simulink model "Linear_and_non_Linear"  (R2024a)
settings: Solver=VariableStepAuto  StartTime=0.0  StopTime=10.0  RelTol=1e-3
values from neighbouring files (symbols this model uses):
  J = (m/12)*(l^2*cos(beta)^2+d^2*sin(beta)^2+w^2)    [Group10_Final_Code_Summer.m]    (also in Group10_Final_Main_Code_Winter.m)
  Kd = 5    [Group10_Final_Code_Summer.m]    (also in Group10_Final_Main_Code_Winter.m)
  Kf = 0.07    [Group10_Final_Code_Summer.m]    (also in Group10_Final_Main_Code_Winter.m)
  Kg = 3000    [Group10_Final_Code_Summer.m]    (also in Group10_Final_Main_Code_Winter.m)
  Kp = 0.318    [Group10_Final_Code_Summer.m]    (also in Group10_Final_Main_Code_Winter.m)
  Kt = 0.07    [Group10_Final_Code_Summer.m]    (also in Group10_Final_Main_Code_Winter.m)
  L = 1e-5    (= 1e-05)    [Group10_Final_Code_Summer.m]    (also in Group10_Final_Main_Code_Winter.m)
  R = 10    [Group10_Final_Code_Summer.m]    (also in Group10_Final_Main_Code_Winter.m)
libraries: simulink x2
settings Model: Creator=marin  LastModifiedBy=marin

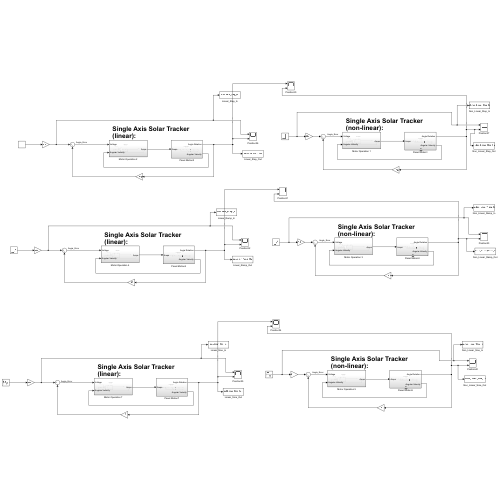
[thumbnail: Simulink's stored preview of the top-level diagram]
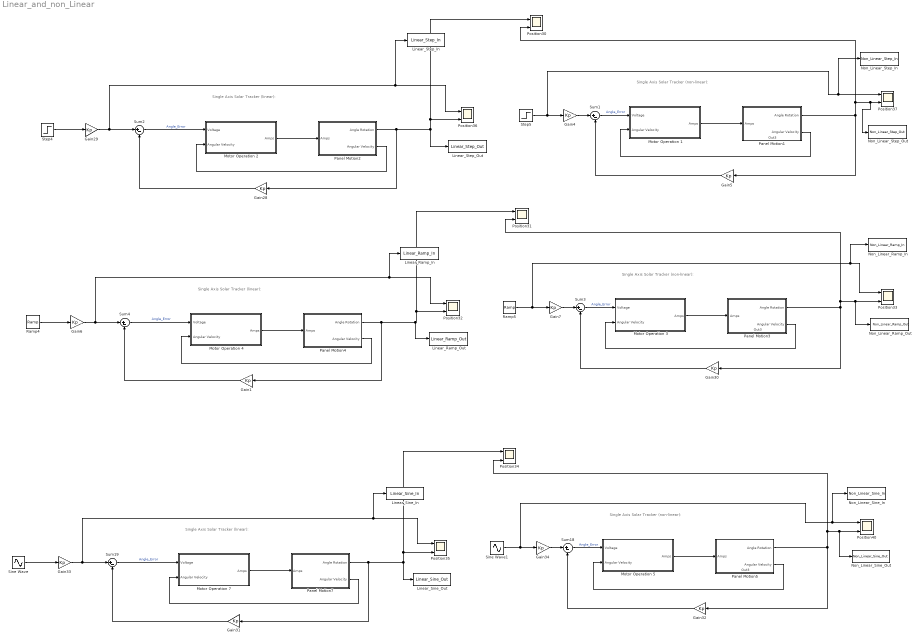
== system Linear_and_non_Linear ==
  note: Single Axis Solar Tracker (linear):
  note: Single Axis Solar Tracker (non-linear):
  note: Single Axis Solar Tracker (non-linear):
  note: Single Axis Solar Tracker (linear):
  note: Single Axis Solar Tracker (linear):
  note: Single Axis Solar Tracker (non-linear):
  Gain{1,4..7,28..34} (12 alike) : Gain  Gain=Kp
  Linear_Ramp_In : ToWorkspace  VariableName=Linear_Ramp_In  SampleTime=-1
  Linear_Ramp_Out : ToWorkspace  VariableName=Linear_Ramp_Out  SampleTime=-1
  Linear_Sine_In : ToWorkspace  VariableName=Linear_Sine_In  SampleTime=-1
  Linear_Sine_Out : ToWorkspace  VariableName=Linear_Sine_Out  SampleTime=-1
  Linear_Step_In : ToWorkspace  VariableName=Linear_Step_In  SampleTime=-1
  Linear_Step_Out : ToWorkspace  VariableName=Linear_Step_Out  SampleTime=-1
  Motor Operation 1 : Subsystem
  Motor Operation 2 : Subsystem
  Motor Operation 3 : Subsystem
  Motor Operation 4 : Subsystem
  Motor Operation 5 : Subsystem
  Motor Operation 7 : Subsystem
  Non_Linear_Ramp_In : ToWorkspace  VariableName=Non_Linear_Ramp_In  SampleTime=-1
  Non_Linear_Ramp_Out : ToWorkspace  VariableName=Non_Linear_Ramp_Out  SampleTime=-1
  Non_Linear_Sine_In : ToWorkspace  VariableName=Non_Linear_Sine_In  SampleTime=-1
  Non_Linear_Sine_Out : ToWorkspace  VariableName=Non_Linear_Sine_Out  SampleTime=-1
  Non_Linear_Step_In : ToWorkspace  VariableName=Non_Linear_Step_In  SampleTime=-1
  Non_Linear_Step_Out : ToWorkspace  VariableName=Non_Linear_Step_Out  SampleTime=-1
  Panel Motion1 : Subsystem
      settings: PortSchema="{\"entries\":[{\"content\":{\"sides\":[{\"content\":{\"connectorIds\":[\"In1\"]},\"type\":\"ConnectorPlacement.EquallySpacedRectSide\",\"uuid\":\"2457b36d-120e-47c4-8d07-640228e5254c\"},{\"content\":{\"connectorIds\":[\"Out1\",\"Out2\"],\"side\":\"RIGHT\"},\"type\":\"ConnectorPlacement.EquallySpacedRectSide\",\"uuid\":\"6776e127-0c13-4a8c-90f1-5ee416f8d651\"},{\"content\":{\"side\":\"TOP\"},\"type\":\"ConnectorPlacement.EquallySpacedRectSide\",\"uuid\":\"01b9375e-d925-43aa-a25a-e625cef73585\"},{\"content\":{\"connectorIds\":[\"Out3\"],\"side\":\"BOTTOM\"},\"type\":\"ConnectorPlacement.EquallySpacedRectSide\",\"uuid\":\"1c8ea06a-a2a0-431e-a15c-ce5bb09036e2\"}]},\"type\":\"ConnectorPlacement.EquallySpacedConnector\",\"uuid\":\"822e0018-41fd-4060-98ab-75615cafefb9\"}],\"packageUris\":[\"http://schema.mathworks.com/mf0/Connector/R2020b\"],\"version\":\"1.0\"}"
  Panel Motion2 : Subsystem
  Panel Motion3 : Subsystem
      settings: PortSchema="{\"entries\":[{\"content\":{\"sides\":[{\"content\":{\"connectorIds\":[\"In1\"]},\"type\":\"ConnectorPlacement.EquallySpacedRectSide\",\"uuid\":\"2457b36d-120e-47c4-8d07-640228e5254c\"},{\"content\":{\"connectorIds\":[\"Out1\",\"Out2\"],\"side\":\"RIGHT\"},\"type\":\"ConnectorPlacement.EquallySpacedRectSide\",\"uuid\":\"6776e127-0c13-4a8c-90f1-5ee416f8d651\"},{\"content\":{\"side\":\"TOP\"},\"type\":\"ConnectorPlacement.EquallySpacedRectSide\",\"uuid\":\"01b9375e-d925-43aa-a25a-e625cef73585\"},{\"content\":{\"connectorIds\":[\"Out3\"],\"side\":\"BOTTOM\"},\"type\":\"ConnectorPlacement.EquallySpacedRectSide\",\"uuid\":\"1c8ea06a-a2a0-431e-a15c-ce5bb09036e2\"}]},\"type\":\"ConnectorPlacement.EquallySpacedConnector\",\"uuid\":\"822e0018-41fd-4060-98ab-75615cafefb9\"}],\"packageUris\":[\"http://schema.mathworks.com/mf0/Connector/R2020b\"],\"version\":\"1.0\"}"
  Panel Motion4 : Subsystem
  Panel Motion5 : Subsystem
      settings: PortSchema="{\"entries\":[{\"content\":{\"sides\":[{\"content\":{\"connectorIds\":[\"In1\"]},\"type\":\"ConnectorPlacement.EquallySpacedRectSide\",\"uuid\":\"2457b36d-120e-47c4-8d07-640228e5254c\"},{\"content\":{\"connectorIds\":[\"Out1\",\"Out2\"],\"side\":\"RIGHT\"},\"type\":\"ConnectorPlacement.EquallySpacedRectSide\",\"uuid\":\"6776e127-0c13-4a8c-90f1-5ee416f8d651\"},{\"content\":{\"side\":\"TOP\"},\"type\":\"ConnectorPlacement.EquallySpacedRectSide\",\"uuid\":\"01b9375e-d925-43aa-a25a-e625cef73585\"},{\"content\":{\"connectorIds\":[\"Out3\"],\"side\":\"BOTTOM\"},\"type\":\"ConnectorPlacement.EquallySpacedRectSide\",\"uuid\":\"1c8ea06a-a2a0-431e-a15c-ce5bb09036e2\"}]},\"type\":\"ConnectorPlacement.EquallySpacedConnector\",\"uuid\":\"822e0018-41fd-4060-98ab-75615cafefb9\"}],\"packageUris\":[\"http://schema.mathworks.com/mf0/Connector/R2020b\"],\"version\":\"1.0\"}"
  Panel Motion7 : Subsystem
  Position{30..37,40} (9 alike) : Scope  NumInputPorts=2
  Ramp4 : simulink/Sources/Ramp  slope=1  start=0  InitialOutput=0
  Ramp5 : simulink/Sources/Ramp  slope=1  start=0  InitialOutput=0
  Sine Wave : Sin  SampleTime=0
  Sine Wave1 : Sin  SampleTime=0
  Step4 : Step  SampleTime=0
  Step5 : Step  SampleTime=0
  Sum{1..4,18..19} (6 alike) : Sum  Inputs=|+-
  wires:
  Sum4/1 -> Motor Operation 4/1(Voltage)  "Angle_Error"
  Ramp4/1 -> Gain6/1
  Sum2/1 -> Motor Operation 2/1(Voltage)  "Angle_Error"
  Sine Wave1/1 -> Non_Linear_Sine_In/1, Position40/1, Gain34/1
  Sum19/1 -> Motor Operation 7/1(Voltage)  "Angle_Error"
  Step5/1 -> Non_Linear_Step_In/1, Position37/1, Gain4/1
  Sine Wave/1 -> Gain33/1
  Sum3/1 -> Motor Operation 3/1(Voltage)  "Angle_Error"
  Panel Motion1/2(Angular Velocity) -> Motor Operation 1/2(Angular Velocity)
  Ramp5/1 -> Gain7/1, Non_Linear_Ramp_In/1, Position33/1
  Gain1/1 -> Sum4/2
  Gain7/1 -> Sum3/1
  Motor Operation 1/1(Amps) -> Panel Motion1/1(Amps)
  Gain5/1 -> Sum1/2
  Gain4/1 -> Sum1/1
  Panel Motion3/1(Angle Rotation) -> Position31/2, Non_Linear_Ramp_Out/1, Position33/2, Gain30/1
  Panel Motion1/1(Angle Rotation) -> Gain5/1, Position30/2, Non_Linear_Step_Out/1, Position37/2
  Gain29/1 -> Sum2/1, Linear_Step_In/1, Position36/1
  Panel Motion4/2(Angular Velocity) -> Motor Operation 4/2(Angular Velocity)
  Sum18/1 -> Motor Operation 5/1(Voltage)  "Angle_Error"
  Panel Motion4/1(Angle Rotation) -> Linear_Ramp_Out/1, Position32/2, Position31/1, Gain1/1
  Panel Motion5/1(Angle Rotation) -> Gain32/1, Position34/2, Non_Linear_Sine_Out/1, Position40/2
  Panel Motion2/1(Angle Rotation) -> Gain28/1, Position30/1, Position36/2, Linear_Step_Out/1
  Motor Operation 2/1(Amps) -> Panel Motion2/1(Amps)
  Panel Motion3/2(Angular Velocity) -> Motor Operation 3/2(Angular Velocity)
  Panel Motion7/2(Angular Velocity) -> Motor Operation 7/2(Angular Velocity)
  Motor Operation 3/1(Amps) -> Panel Motion3/1(Amps)
  Motor Operation 7/1(Amps) -> Panel Motion7/1(Amps)
  Gain34/1 -> Sum18/1
  Gain6/1 -> Linear_Ramp_In/1, Position32/1, Sum4/1
  Panel Motion5/2(Angular Velocity) -> Motor Operation 5/2(Angular Velocity)
  Gain32/1 -> Sum18/2
  Motor Operation 4/1(Amps) -> Panel Motion4/1(Amps)
  Step4/1 -> Gain29/1
  Gain31/1 -> Sum19/2
  Sum1/1 -> Motor Operation 1/1(Voltage)  "Angle_Error"
  Motor Operation 5/1(Amps) -> Panel Motion5/1(Amps)
  Gain28/1 -> Sum2/2
  Gain33/1 -> Sum19/1, Linear_Sine_In/1, Position35/1
  Panel Motion2/2(Angular Velocity) -> Motor Operation 2/2(Angular Velocity)
  Gain30/1 -> Sum3/2
  Panel Motion7/1(Angle Rotation) -> Gain31/1, Linear_Sine_Out/1, Position34/1, Position35/2

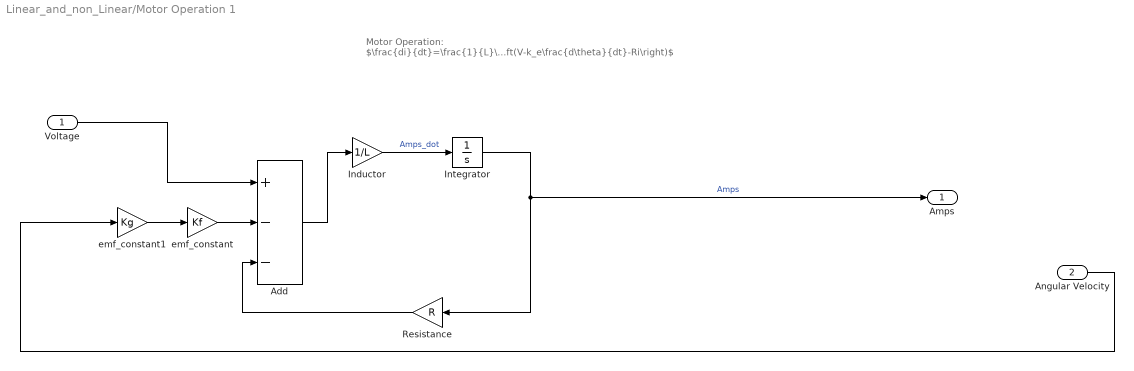
== system Linear_and_non_Linear/Motor Operation 1 ==
  note: Motor Operation:
      | $\frac{di}{dt}=\frac{1}{L}\left(V-k_e\frac{d\theta}{dt}-Ri\right)$
  Voltage : Inport
  Angular Velocity : Inport  Port=2
  Add : Sum  Inputs=+--
  Inductor : Gain  Gain=1/L
  Integrator : Integrator
  Resistance : Gain  Gain=R
  emf_constant : Gain  Gain=Kf
  emf_constant1 : Gain  Gain=Kg
  Amps : Outport
  wires:
  emf_constant/1 -> Add/2
  Resistance/1 -> Add/3
  Add/1 -> Inductor/1
  Inductor/1 -> Integrator/1  "Amps_dot"
  Angular Velocity/1 -> emf_constant1/1
  Voltage/1 -> Add/1
  Integrator/1 -> Resistance/1, Amps/1  "Amps"
  emf_constant1/1 -> emf_constant/1

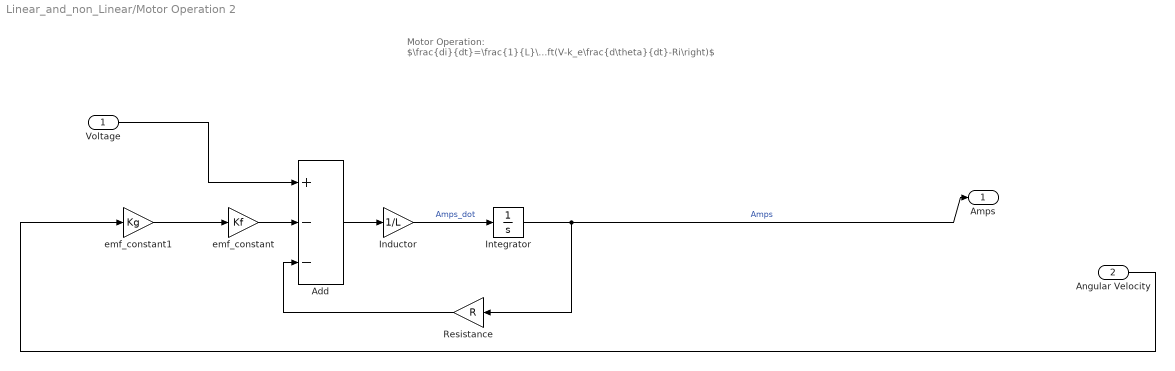
== system Linear_and_non_Linear/Motor Operation 2 ==
  note: Motor Operation:
      | $\frac{di}{dt}=\frac{1}{L}\left(V-k_e\frac{d\theta}{dt}-Ri\right)$
  Voltage : Inport
  Angular Velocity : Inport  Port=2
  Add : Sum  Inputs=+--
  Inductor : Gain  Gain=1/L
  Integrator : Integrator
  Resistance : Gain  Gain=R
  emf_constant : Gain  Gain=Kf
  emf_constant1 : Gain  Gain=Kg
  Amps : Outport
  wires:
  emf_constant/1 -> Add/2
  Resistance/1 -> Add/3
  Add/1 -> Inductor/1
  Inductor/1 -> Integrator/1  "Amps_dot"
  Angular Velocity/1 -> emf_constant1/1
  Voltage/1 -> Add/1
  Integrator/1 -> Amps/1, Resistance/1  "Amps"
  emf_constant1/1 -> emf_constant/1

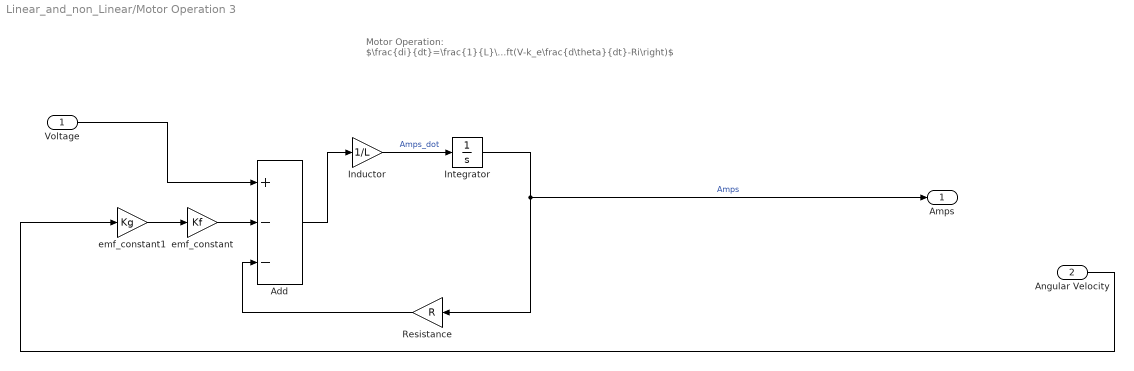
== system Linear_and_non_Linear/Motor Operation 3 ==
  note: Motor Operation:
      | $\frac{di}{dt}=\frac{1}{L}\left(V-k_e\frac{d\theta}{dt}-Ri\right)$
  Voltage : Inport
  Angular Velocity : Inport  Port=2
  Add : Sum  Inputs=+--
  Inductor : Gain  Gain=1/L
  Integrator : Integrator
  Resistance : Gain  Gain=R
  emf_constant : Gain  Gain=Kf
  emf_constant1 : Gain  Gain=Kg
  Amps : Outport
  wires:
  emf_constant1/1 -> emf_constant/1
  Integrator/1 -> Amps/1, Resistance/1  "Amps"
  Voltage/1 -> Add/1
  Angular Velocity/1 -> emf_constant1/1
  Inductor/1 -> Integrator/1  "Amps_dot"
  Add/1 -> Inductor/1
  Resistance/1 -> Add/3
  emf_constant/1 -> Add/2

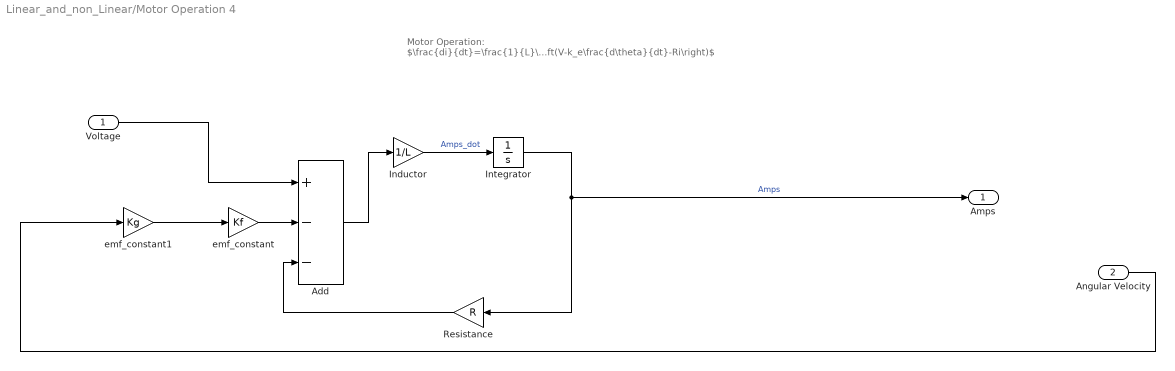
== system Linear_and_non_Linear/Motor Operation 4 ==
  note: Motor Operation:
      | $\frac{di}{dt}=\frac{1}{L}\left(V-k_e\frac{d\theta}{dt}-Ri\right)$
  Voltage : Inport
  Angular Velocity : Inport  Port=2
  Add : Sum  Inputs=+--
  Inductor : Gain  Gain=1/L
  Integrator : Integrator
  Resistance : Gain  Gain=R
  emf_constant : Gain  Gain=Kf
  emf_constant1 : Gain  Gain=Kg
  Amps : Outport
  wires:
  emf_constant1/1 -> emf_constant/1
  Integrator/1 -> Amps/1, Resistance/1  "Amps"
  Voltage/1 -> Add/1
  Angular Velocity/1 -> emf_constant1/1
  Inductor/1 -> Integrator/1  "Amps_dot"
  Add/1 -> Inductor/1
  Resistance/1 -> Add/3
  emf_constant/1 -> Add/2

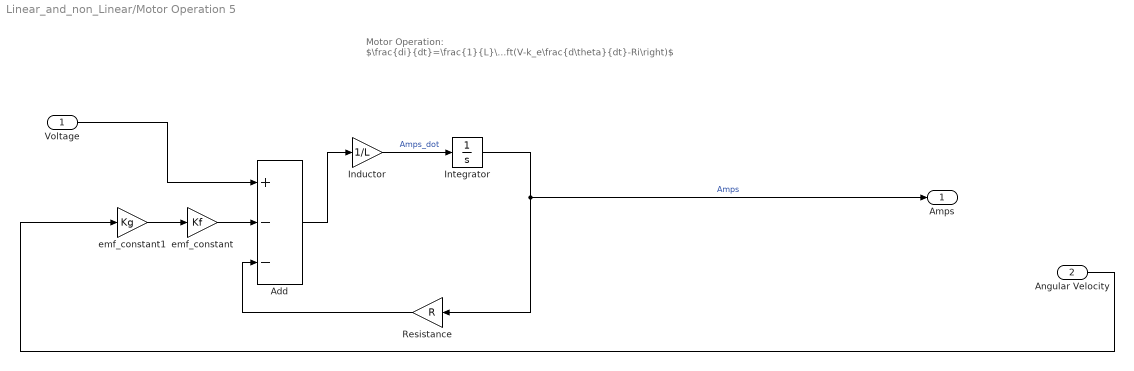
== system Linear_and_non_Linear/Motor Operation 5 ==
  note: Motor Operation:
      | $\frac{di}{dt}=\frac{1}{L}\left(V-k_e\frac{d\theta}{dt}-Ri\right)$
  Voltage : Inport
  Angular Velocity : Inport  Port=2
  Add : Sum  Inputs=+--
  Inductor : Gain  Gain=1/L
  Integrator : Integrator
  Resistance : Gain  Gain=R
  emf_constant : Gain  Gain=Kf
  emf_constant1 : Gain  Gain=Kg
  Amps : Outport
  wires:
  emf_constant/1 -> Add/2
  Resistance/1 -> Add/3
  Add/1 -> Inductor/1
  Inductor/1 -> Integrator/1  "Amps_dot"
  Angular Velocity/1 -> emf_constant1/1
  Voltage/1 -> Add/1
  Integrator/1 -> Resistance/1, Amps/1  "Amps"
  emf_constant1/1 -> emf_constant/1

== system Linear_and_non_Linear/Motor Operation 7 ==
  note: Motor Operation:
      | $\frac{di}{dt}=\frac{1}{L}\left(V-k_e\frac{d\theta}{dt}-Ri\right)$
  Voltage : Inport
  Angular Velocity : Inport  Port=2
  Add : Sum  Inputs=+--
  Inductor : Gain  Gain=1/L
  Integrator : Integrator
  Resistance : Gain  Gain=R
  emf_constant : Gain  Gain=Kf
  emf_constant1 : Gain  Gain=Kg
  Amps : Outport
  wires:
  emf_constant/1 -> Add/2
  Resistance/1 -> Add/3
  Add/1 -> Inductor/1
  Inductor/1 -> Integrator/1  "Amps_dot"
  Angular Velocity/1 -> emf_constant1/1
  Voltage/1 -> Add/1
  Integrator/1 -> Resistance/1, Amps/1  "Amps"
  emf_constant1/1 -> emf_constant/1

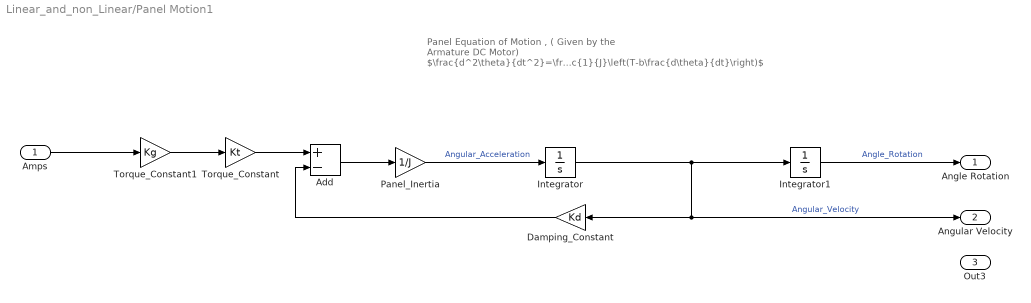
== system Linear_and_non_Linear/Panel Motion1 ==
  note: Panel Equation of Motion ,
      | ( Given by the Armature DC Motor)
      | $\frac{d^2\theta}{dt^2}=\frac{1}{J}\left(T-b\frac{d\theta}{dt}\right)$
  Amps : Inport
  Add : Sum  Inputs=+-
  Damping_Constant : Gain  Gain=Kd
  Integrator : Integrator
  Integrator1 : Integrator
  Panel_Inertia : Gain  Gain=1/J
  Torque_Constant : Gain  Gain=Kt
  Torque_Constant1 : Gain  Gain=Kg
  Angle Rotation : Outport
  Angular Velocity : Outport  Port=2
  Out3 : Outport  Port=3
  wires:
  Integrator1/1 -> Angle Rotation/1  "Angle_Rotation"
  Panel_Inertia/1 -> Integrator/1  "Angular_Acceleration"
  Amps/1 -> Torque_Constant1/1
  Add/1 -> Panel_Inertia/1
  Damping_Constant/1 -> Add/2
  Integrator/1 -> Angular Velocity/1, Damping_Constant/1, Integrator1/1  "Angular_Velocity"
  Torque_Constant/1 -> Add/1
  Torque_Constant1/1 -> Torque_Constant/1

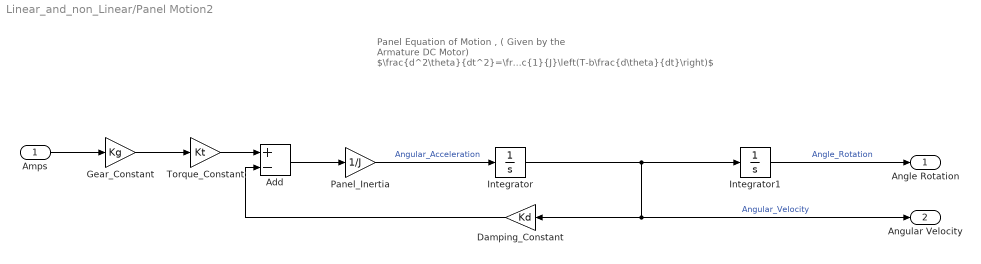
== system Linear_and_non_Linear/Panel Motion2 ==
  note: Panel Equation of Motion ,
      | ( Given by the Armature DC Motor)
      | $\frac{d^2\theta}{dt^2}=\frac{1}{J}\left(T-b\frac{d\theta}{dt}\right)$
  Amps : Inport
  Add : Sum  Inputs=+-
  Damping_Constant : Gain  Gain=Kd
  Gear_Constant : Gain  Gain=Kg
  Integrator : Integrator
  Integrator1 : Integrator
  Panel_Inertia : Gain  Gain=1/J
  Torque_Constant : Gain  Gain=Kt
  Angle Rotation : Outport
  Angular Velocity : Outport  Port=2
  wires:
  Integrator1/1 -> Angle Rotation/1  "Angle_Rotation"
  Panel_Inertia/1 -> Integrator/1  "Angular_Acceleration"
  Amps/1 -> Gear_Constant/1
  Add/1 -> Panel_Inertia/1
  Damping_Constant/1 -> Add/2
  Integrator/1 -> Angular Velocity/1, Damping_Constant/1, Integrator1/1  "Angular_Velocity"
  Torque_Constant/1 -> Add/1
  Gear_Constant/1 -> Torque_Constant/1

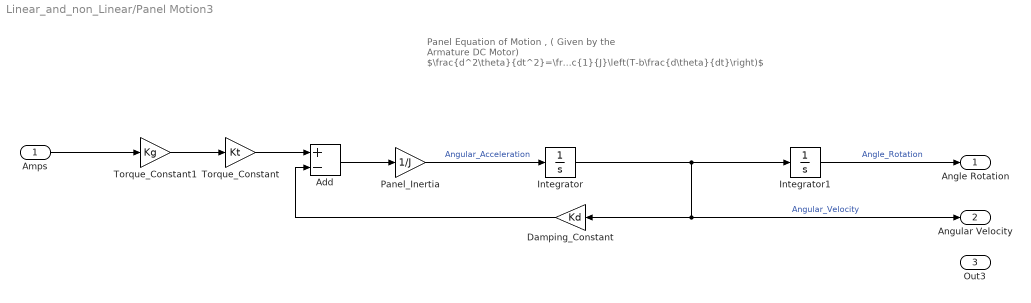
== system Linear_and_non_Linear/Panel Motion3 ==
  note: Panel Equation of Motion ,
      | ( Given by the Armature DC Motor)
      | $\frac{d^2\theta}{dt^2}=\frac{1}{J}\left(T-b\frac{d\theta}{dt}\right)$
  Amps : Inport
  Add : Sum  Inputs=+-
  Damping_Constant : Gain  Gain=Kd
  Integrator : Integrator
  Integrator1 : Integrator
  Panel_Inertia : Gain  Gain=1/J
  Torque_Constant : Gain  Gain=Kt
  Torque_Constant1 : Gain  Gain=Kg
  Angle Rotation : Outport
  Angular Velocity : Outport  Port=2
  Out3 : Outport  Port=3
  wires:
  Torque_Constant1/1 -> Torque_Constant/1
  Torque_Constant/1 -> Add/1
  Integrator/1 -> Integrator1/1, Damping_Constant/1, Angular Velocity/1  "Angular_Velocity"
  Damping_Constant/1 -> Add/2
  Add/1 -> Panel_Inertia/1
  Amps/1 -> Torque_Constant1/1
  Panel_Inertia/1 -> Integrator/1  "Angular_Acceleration"
  Integrator1/1 -> Angle Rotation/1  "Angle_Rotation"

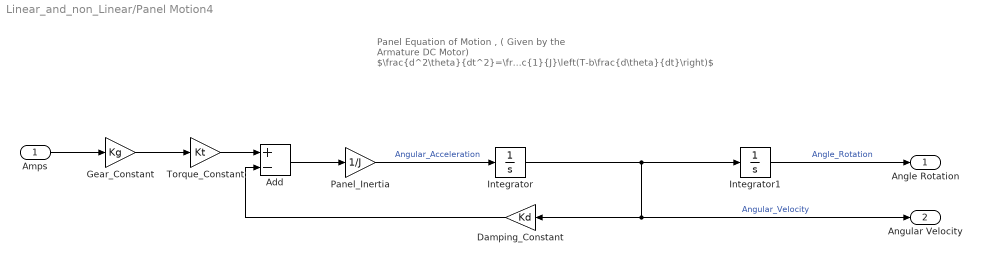
== system Linear_and_non_Linear/Panel Motion4 ==
  note: Panel Equation of Motion ,
      | ( Given by the Armature DC Motor)
      | $\frac{d^2\theta}{dt^2}=\frac{1}{J}\left(T-b\frac{d\theta}{dt}\right)$
  Amps : Inport
  Add : Sum  Inputs=+-
  Damping_Constant : Gain  Gain=Kd
  Gear_Constant : Gain  Gain=Kg
  Integrator : Integrator
  Integrator1 : Integrator
  Panel_Inertia : Gain  Gain=1/J
  Torque_Constant : Gain  Gain=Kt
  Angle Rotation : Outport
  Angular Velocity : Outport  Port=2
  wires:
  Gear_Constant/1 -> Torque_Constant/1
  Torque_Constant/1 -> Add/1
  Integrator/1 -> Integrator1/1, Damping_Constant/1, Angular Velocity/1  "Angular_Velocity"
  Damping_Constant/1 -> Add/2
  Add/1 -> Panel_Inertia/1
  Amps/1 -> Gear_Constant/1
  Panel_Inertia/1 -> Integrator/1  "Angular_Acceleration"
  Integrator1/1 -> Angle Rotation/1  "Angle_Rotation"

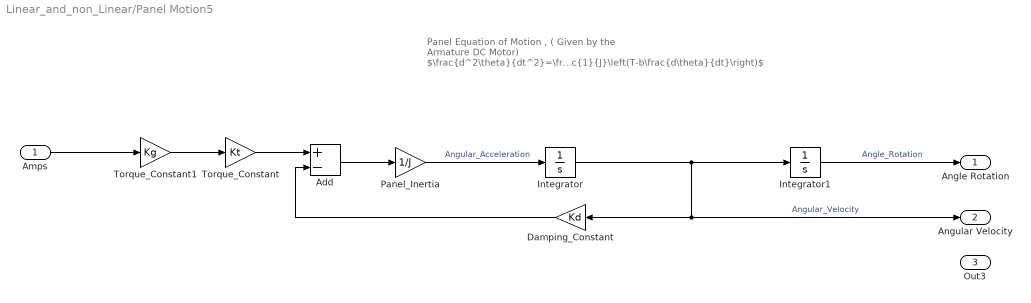
== system Linear_and_non_Linear/Panel Motion5 ==
  note: Panel Equation of Motion ,
      | ( Given by the Armature DC Motor)
      | $\frac{d^2\theta}{dt^2}=\frac{1}{J}\left(T-b\frac{d\theta}{dt}\right)$
  Amps : Inport
  Add : Sum  Inputs=+-
  Damping_Constant : Gain  Gain=Kd
  Integrator : Integrator
  Integrator1 : Integrator
  Panel_Inertia : Gain  Gain=1/J
  Torque_Constant : Gain  Gain=Kt
  Torque_Constant1 : Gain  Gain=Kg
  Angle Rotation : Outport
  Angular Velocity : Outport  Port=2
  Out3 : Outport  Port=3
  wires:
  Integrator1/1 -> Angle Rotation/1  "Angle_Rotation"
  Panel_Inertia/1 -> Integrator/1  "Angular_Acceleration"
  Amps/1 -> Torque_Constant1/1
  Add/1 -> Panel_Inertia/1
  Damping_Constant/1 -> Add/2
  Integrator/1 -> Angular Velocity/1, Damping_Constant/1, Integrator1/1  "Angular_Velocity"
  Torque_Constant/1 -> Add/1
  Torque_Constant1/1 -> Torque_Constant/1

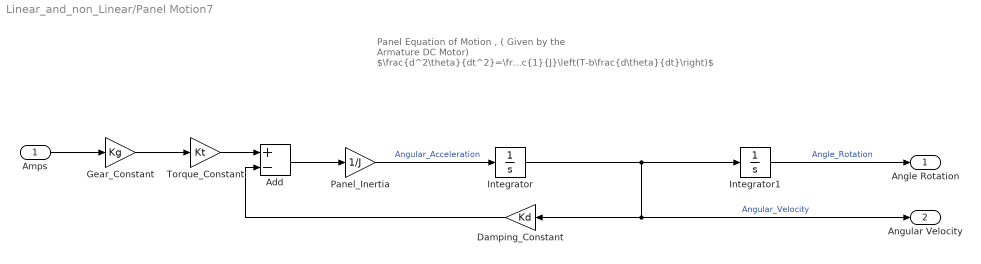
== system Linear_and_non_Linear/Panel Motion7 ==
  note: Panel Equation of Motion ,
      | ( Given by the Armature DC Motor)
      | $\frac{d^2\theta}{dt^2}=\frac{1}{J}\left(T-b\frac{d\theta}{dt}\right)$
  Amps : Inport
  Add : Sum  Inputs=+-
  Damping_Constant : Gain  Gain=Kd
  Gear_Constant : Gain  Gain=Kg
  Integrator : Integrator
  Integrator1 : Integrator
  Panel_Inertia : Gain  Gain=1/J
  Torque_Constant : Gain  Gain=Kt
  Angle Rotation : Outport
  Angular Velocity : Outport  Port=2
  wires:
  Integrator1/1 -> Angle Rotation/1  "Angle_Rotation"
  Panel_Inertia/1 -> Integrator/1  "Angular_Acceleration"
  Amps/1 -> Gear_Constant/1
  Add/1 -> Panel_Inertia/1
  Damping_Constant/1 -> Add/2
  Integrator/1 -> Angular Velocity/1, Damping_Constant/1, Integrator1/1  "Angular_Velocity"
  Torque_Constant/1 -> Add/1
  Gear_Constant/1 -> Torque_Constant/1
